simulink model "tanks_demo_2"  (Simulink 9.2)
settings: Solver=VariableStepAuto  StartTime=0.0  StopTime=10.0  RelTol=1e-3
values from neighbouring files (symbols this model uses):
  C = sysDis.C    [control_design.m]
  Gamma = sysDis.B    [control_design.m]
  L = acker(Phi,Gamma,p_controller)    [control_design.m]
  lr = num / den    [control_design.m]
  M = acker(Phi',C',p_observer)    [control_design.m]
  Phi = sysDis.A    [control_design.m]
  Ts = 4    [control_design.m]
  uss = alpha2/beta*sqrt(2*g*tank_init_h2)*100/15    [control_design.m]
  yss = 40    [control_design.m]
undefined symbols (not defined in the file or in its folder): tank_A1, tank_a1, tank_A2, tank_a2, tank_H1, tank_H2, tank_init_h1, tank_init_h2, tank_Kpump
settings Model: Creator=srirama  LastModifiedBy=srirama
settings DataIOCC: LimitDataPoints=off  SaveFormat=Dataset  SignalLoggingSaveFormat=Dataset
settings OptimizationCC: LifeSpan=auto
settings DebuggingCC: UnderspecifiedInitializationDetection=Simplified  MergeDetectMultiDrivingBlocksExec=error  FcnCallInpInsideContextMsg=error  StateNameClashWarn=none  SFUnexpectedBacktrackingDiag=error  SFNoUnconditionalDefaultTransitionDiag=error  SFExecutionAtInitializationDiag=warning
settings HardwareCC: ProdBitPerPointer=64  ProdBitPerSizeT=64  ProdBitPerPtrDiffT=64  ProdLargestAtomicFloat=Float  ProdIntDivRoundTo=Zero  ProdEndianess=LittleEndian  ProdWordSize=64  ProdHWDeviceType=Intel->x86-64 (Windows64)
settings ModelReferenceCC: PropagateSignalLabelsOutOfModel=on
settings SFSimCC: SimUseLocalCustomCode=on
settings RTWCC: RTWUseLocalCustomCode=on
settings CodeAppCC: StateflowObjectComments=off
settings GRTTargetCC: TargetLangStandard=C99 (ISO)  GeneratePreprocessorConditionals=Use local settings  CombineOutputUpdateFcns=on  GRTInterface=off
settings ConfigComp: CovMetricSettings=dwe  CovHtmlReporting=off  CovSaveCumulativeToWorkspaceVar=off  CovSaveSingleToWorkspaceVar=off  CovExternalEMLEnable=on

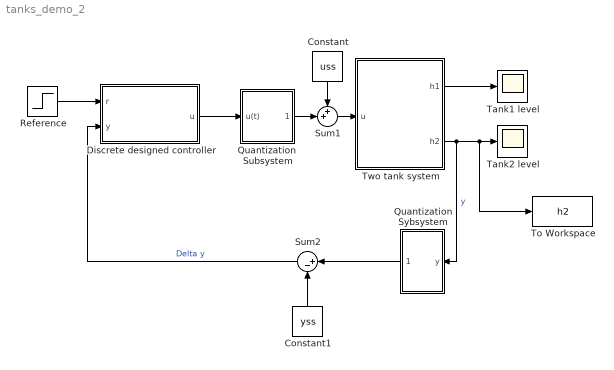
== system tanks_demo_2 ==
  Constant : Constant  Value=uss
  Constant1 : Constant  Value=yss
  Discrete designed controller : Subsystem
  Quantization Sybsystem : Subsystem
  Quantization  Subsystem : Subsystem
  Reference : Step  Time=25  After=10  SampleTime=0
  Sum1 : Sum  Inputs=++|
  Sum2 : Sum  Inputs=|+-
  Tank1 level : Scope
  Tank2 level : Scope
  To Workspace : ToWorkspace  VariableName=h2  SaveFormat=Timeseries  SampleTime=-1
  Two tank system : Subsystem
  wires:
  Sum1/1 -> Two tank system/1(u)
  Reference/1 -> Discrete designed controller/1(r)
  Constant1/1 -> Sum2/2
  Two tank system/1(h1) -> Tank1 level/1
  Sum2/1 -> Discrete designed controller/2(y)  "Delta y"
  Two tank system/2(h2) -> To Workspace/1, Tank2 level/1, Quantization Sybsystem/1(y)  "y"
  Constant/1 -> Sum1/1
  Discrete designed controller/1(u) -> Quantization  Subsystem/1(u(t))
  Quantization  Subsystem/1(uQ(t)) -> Sum1/2
  Quantization Sybsystem/1(yQ(t)) -> Sum2/1

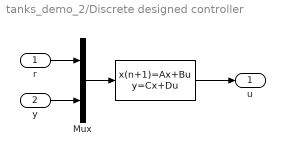
== system tanks_demo_2/Discrete designed controller ==
  r : Inport
  y : Inport  Port=2
  "   " : DiscreteStateSpace  A=Phi-Gamma*L-M'*C  B=[lr .* Gamma M']  C=-L  D=[lr 0]  SampleTime=Ts
  Mux : Mux  Inputs=2
  u : Outport
  wires:
  "   "/1 -> u/1
  Mux/1 -> "   "/1
  y/1 -> Mux/2
  r/1 -> Mux/1

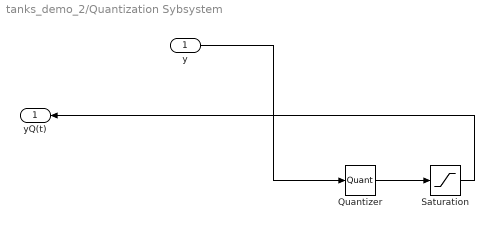
== system tanks_demo_2/Quantization Sybsystem ==
  y : Inport
  Quantizer : Quantizer  QuantizationInterval=Qt
  Saturation : Saturate  UpperLimit=100  LowerLimit=0
  yQ(t) : Outport
  wires:
  Quantizer/1 -> Saturation/1
  y/1 -> Quantizer/1
  Saturation/1 -> yQ(t)/1

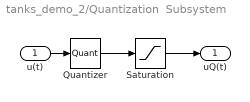
== system tanks_demo_2/Quantization  Subsystem ==
  u(t) : Inport
  Quantizer : Quantizer  QuantizationInterval=Qt
  Saturation : Saturate  UpperLimit=100  LowerLimit=0
  uQ(t) : Outport
  wires:
  Saturation/1 -> uQ(t)/1
  u(t)/1 -> Quantizer/1
  Quantizer/1 -> Saturation/1

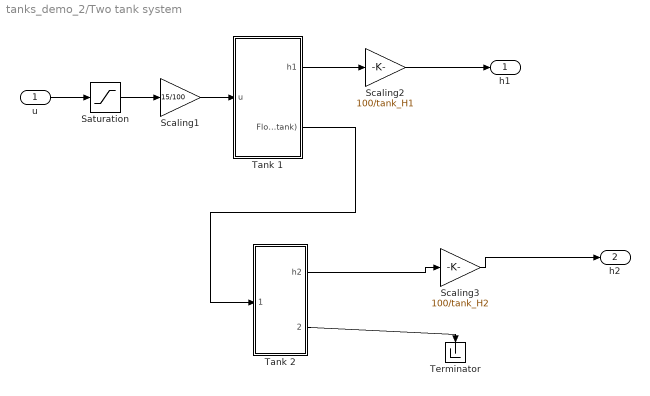
== system tanks_demo_2/Two tank system ==
  u : Inport
  Saturation : Saturate  UpperLimit=100  LowerLimit=-0
  Scaling1 : Gain  Gain=15/100  SaturateOnIntegerOverflow=on  OutDataTypeStr=Inherit: Same as input  ParamDataTypeStr=Inherit: Same as input
  Scaling2 : Gain  Gain=100/tank_H1  SaturateOnIntegerOverflow=on  OutDataTypeStr=Inherit: Same as input  ParamDataTypeStr=Inherit: Same as input
  Scaling3 : Gain  Gain=100/tank_H2  SaturateOnIntegerOverflow=on  OutDataTypeStr=Inherit: Same as input  ParamDataTypeStr=Inherit: Same as input
  Tank 1 : Subsystem
  Tank 2 : Subsystem
  Terminator : Terminator
  h1 : Outport
  h2 : Outport  Port=2
  wires:
  Tank 2/1(h2) -> Scaling3/1
  Tank 2/2(Flow out) -> Terminator/1
  u/1 -> Saturation/1
  Tank 1/1(h1) -> Scaling2/1
  Tank 1/2(Flow out  (to lower tank)) -> Tank 2/1(From upper tank)
  Scaling2/1 -> h1/1
  Scaling3/1 -> h2/1
  Scaling1/1 -> Tank 1/1(u)
  Saturation/1 -> Scaling1/1

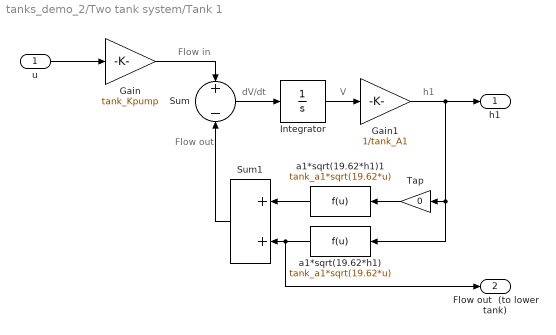
== system tanks_demo_2/Two tank system/Tank 1 ==
  note: h1
  note: V
  note: dV/dt
  note: Flow out
  note: Flow in
  u : Inport
  Gain : Gain  Gain=tank_Kpump  SaturateOnIntegerOverflow=on  OutDataTypeStr=Inherit: Same as input  ParamDataTypeStr=Inherit: Same as input
  Gain1 : Gain  Gain=1/tank_A1  SaturateOnIntegerOverflow=on  OutDataTypeStr=Inherit: Same as input  ParamDataTypeStr=Inherit: Same as input
  Integrator : Integrator  InitialCondition=tank_init_h1*tank_A1  LimitOutput=on  UpperSaturationLimit=tank_H1*tank_A1  LowerSaturationLimit=0
  Sum : Sum  Inputs=+-  SaturateOnIntegerOverflow=on  InputSameDT=on  OutDataTypeStr=Inherit: Same as first input
  Sum1 : Sum  SaturateOnIntegerOverflow=on  InputSameDT=on  OutDataTypeStr=Inherit: Same as first input
  Tap : Gain  Gain=0  SaturateOnIntegerOverflow=on  OutDataTypeStr=Inherit: Same as input  ParamDataTypeStr=Inherit: Same as input
  a1*sqrt(19.62*h1) : Fcn  Expr=tank_a1*sqrt(19.62*u)
  a1*sqrt(19.62*h1)1 : Fcn  Expr=tank_a1*sqrt(19.62*u)
  h1 : Outport
  Flow out  (to lower tank) : Outport  Port=2
  wires:
  Gain1/1 -> Tap/1, a1*sqrt(19.62*h1)/1, h1/1
  Integrator/1 -> Gain1/1
  Sum/1 -> Integrator/1
  Gain/1 -> Sum/1
  u/1 -> Gain/1
  a1*sqrt(19.62*h1)/1 -> Flow out  (to lower tank)/1, Sum1/2
  a1*sqrt(19.62*h1)1/1 -> Sum1/1
  Sum1/1 -> Sum/2
  Tap/1 -> a1*sqrt(19.62*h1)1/1

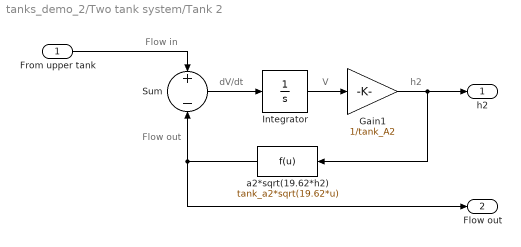
== system tanks_demo_2/Two tank system/Tank 2 ==
  note: Flow in
  note: Flow out
  note: dV/dt
  note: V
  note: h2
  From upper tank : Inport
  Gain1 : Gain  Gain=1/tank_A2  SaturateOnIntegerOverflow=on  OutDataTypeStr=Inherit: Same as input  ParamDataTypeStr=Inherit: Same as input
  Integrator : Integrator  InitialCondition=tank_init_h2*tank_A2  LimitOutput=on  UpperSaturationLimit=tank_H2*tank_A2  LowerSaturationLimit=0
  Sum : Sum  Inputs=+-  SaturateOnIntegerOverflow=on  InputSameDT=on  OutDataTypeStr=Inherit: Same as first input
  a2*sqrt(19.62*h2) : Fcn  Expr=tank_a2*sqrt(19.62*u)
  h2 : Outport
  Flow out : Outport  Port=2
  wires:
  Sum/1 -> Integrator/1
  Integrator/1 -> Gain1/1
  Gain1/1 -> h2/1, a2*sqrt(19.62*h2)/1
  a2*sqrt(19.62*h2)/1 -> Sum/2, Flow out/1
  From upper tank/1 -> Sum/1
